simulink model "czaso_optymal_przyk"  (R2023b)
settings: Solver=FixedStepAuto  StartTime=0.0  StopTime=50  FixedStep=0.01  RelTol=1e-3  EnableMultiTasking=on
values from neighbouring files (symbols this model uses):
  B = Bw(i)    [lab7.m]
  w = 1    [lab7.m]
  x0 = -3    [lab7.m]
  xp0 = 4    [lab7.m]
settings Model: Creator=pc  LastModifiedBy=pc
settings SolverCC: ZeroCrossAlgorithm=Adaptive
settings DataIOCC: LimitDataPoints=on  SaveFormat=Array  SignalLoggingSaveFormat=ModelDataLogs  ReturnWorkspaceOutputs=off  SignalLoggingName=sigsOut
settings OptimizationCC: BooleanDataType=off
settings DebuggingCC: SaveWithParameterizedLinksMsg=none  UnderspecifiedInitializationDetection=Classic  MergeDetectMultiDrivingBlocksExec=none  SignalResolutionControl=TryResolveAllWithWarning  IgnoredZcDiagnostic=none  MultiTaskDSMMsg=warning  MultiTaskCondExecSysMsg=none  UnconnectedInputMsg=warning  UnconnectedOutputMsg=warning  UnconnectedLineMsg=warning
settings HardwareCC: ProdBitPerPointer=32  ProdBitPerSizeT=32  ProdBitPerPtrDiffT=32  ProdLargestAtomicFloat=None  ProdIntDivRoundTo=Undefined  ProdEndianess=Unspecified  ProdWordSize=32  ProdHWDeviceType=32-bit Generic  TargetUnknown=on
settings ModelReferenceCC: PropagateSignalLabelsOutOfModel=off
settings GRTTargetCC: CombineOutputUpdateFcns=off  GRTInterface=on
settings ConfigComp: CovMetricSettings=dw  CovSaveCumulativeToWorkspaceVar=on  CovSaveSingleToWorkspaceVar=on

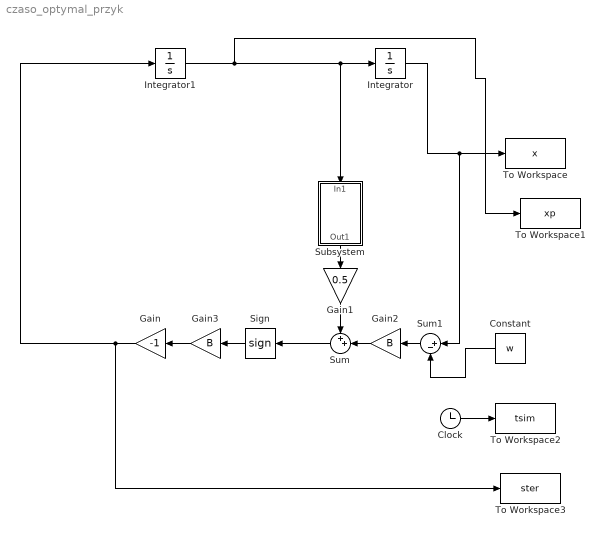
== system czaso_optymal_przyk ==
  Clock : Clock
      settings: Decimation=1000
  Constant : Constant  Value=w
  Gain : Gain  Gain=-1  SaturateOnIntegerOverflow=on  OutDataTypeStr=Inherit: Same as input  ParamDataTypeStr=Inherit: Same as input
  Gain1 : Gain  Gain=0.5  SaturateOnIntegerOverflow=on  OutDataTypeStr=Inherit: Same as input  ParamDataTypeStr=Inherit: Same as input
  Gain2 : Gain  Gain=B
  Gain3 : Gain  Gain=B
  Integrator : Integrator  InitialCondition=xp0
  Integrator1 : Integrator  InitialCondition=x0
  Sign : Signum
  Subsystem : Subsystem
  Sum : Sum  Inputs=++|  InputSameDT=on  SaturateOnIntegerOverflow=on  OutDataTypeStr=Inherit: Same as first input
  Sum1 : Sum  Inputs=|+-
  To Workspace : ToWorkspace  VariableName=x  SampleTime=-1
  To Workspace1 : ToWorkspace  VariableName=xp  SampleTime=-1
  To Workspace2 : ToWorkspace  VariableName=tsim  SampleTime=-1
  To Workspace3 : ToWorkspace  VariableName=ster  SampleTime=-1
  wires:
  Subsystem/1(Out1) -> Gain1/1
  Sum/1 -> Sign/1
  Gain/1 -> Integrator1/1, To Workspace3/1
  Gain1/1 -> Sum/1
  Integrator1/1 -> Integrator/1, Subsystem/1(In1), To Workspace1/1
  Integrator/1 -> Sum1/1, To Workspace/1
  Clock/1 -> To Workspace2/1
  Constant/1 -> Sum1/2
  Gain3/1 -> Gain/1
  Sign/1 -> Gain3/1
  Gain2/1 -> Sum/2
  Sum1/1 -> Gain2/1

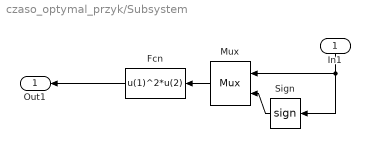
== system czaso_optymal_przyk/Subsystem ==
  In1 : Inport
  Fcn : Fcn  Expr=u(1)^2*u(2)
  Mux : Mux  Inputs=2
      settings: DisplayOption=signals
  Sign : Signum
  Out1 : Outport
  wires:
  Mux/1 -> Fcn/1
  Sign/1 -> Mux/2
  In1/1 -> Sign/1, Mux/1
  Fcn/1 -> Out1/1
